simulink model "differential_drive"  (R2018a)
settings: Solver=FixedStepAuto  StartTime=0.0  StopTime=inf  FixedStep=0.7  RelTol=1e-3
settings Model: EnablePacing=on  Creator=U500304  LastModifiedBy=U500304

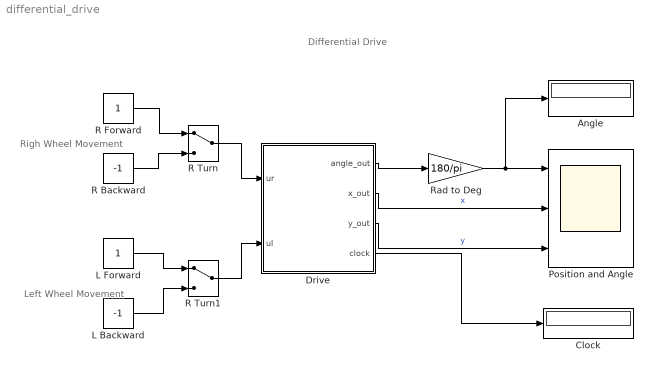
== system differential_drive ==
  note: Righ Wheel
      | Movement
  note: Differential Drive
  note: Left Wheel
      | Movement
  Angle : Display
      settings: AttributesFormatString=Degrees
  Clock : Display
  Drive : Stateflow chart  TreatAsAtomicUnit=on
  L Backward : Constant  Value=-1
  L Forward : Constant
  Position and Angle : Scope  NumInputPorts=3
  R Backward : Constant  Value=-1
  R Forward : Constant
  R Turn : ManualSwitch
  R Turn1 : ManualSwitch
  Rad to Deg : Gain  Gain=180/pi
  wires:
  R Forward/1 -> R Turn/1
  Drive/1(angle_out) -> Rad to Deg/1
  Drive/2(x_out) -> Position and Angle/2  "x"
  Drive/3(y_out) -> Position and Angle/3  "y"
  R Backward/1 -> R Turn/2
  R Turn/1 -> Drive/1(ur)
  L Forward/1 -> R Turn1/1
  L Backward/1 -> R Turn1/2
  R Turn1/1 -> Drive/2(ul)
  Rad to Deg/1 -> Angle/1, Position and Angle/1
  Drive/4(clock) -> Clock/1

== stateflow chart differential_drive/Drive ==
  settings: updateMethod=CONTINUOUS
  state GoForward
    en:
    clock = 0;
    du:
    x_dot = (r / 2) * (ul + ur) * cos(angle);
    y_dot = (r / 2) * (ul + ur) * sin(angle);
    angle_dot = (r / L) * (ur - ul);
    angle_out = angle;
    x_out = x;
    y_out = y;
    clock_dot = 1;
  (default) -> GoForward
  data: ur input; ul input; angle local =0; x local =0; y local =0; r constant double =10; L constant double =100; angle_out output; x_out output; y_out output; clock output =0
  data angle settings: updateMethod=SF_CONTINUOUS_TIME_DATA
  data x settings: updateMethod=SF_CONTINUOUS_TIME_DATA
  data y settings: updateMethod=SF_CONTINUOUS_TIME_DATA
  data clock settings: updateMethod=SF_CONTINUOUS_TIME_DATA
